simulink model "es3_sim"  (Simulink 7.5)
settings: Solver=ode45  StartTime=0.0  StopTime=10.0  RelTol=1e-3
values from neighbouring files (symbols this model uses):
  e_ = 0.1    [es3.m]
  epsilon1 = 40    [es3.m]
  epsilon2 = 10    [es3.m]
  k1 = 800    [es3.m]
  p = 0.2    [es3.m]
libraries: simulink x1
settings Model: Creator=Koldar  LastModifiedBy=ceco-sciallo

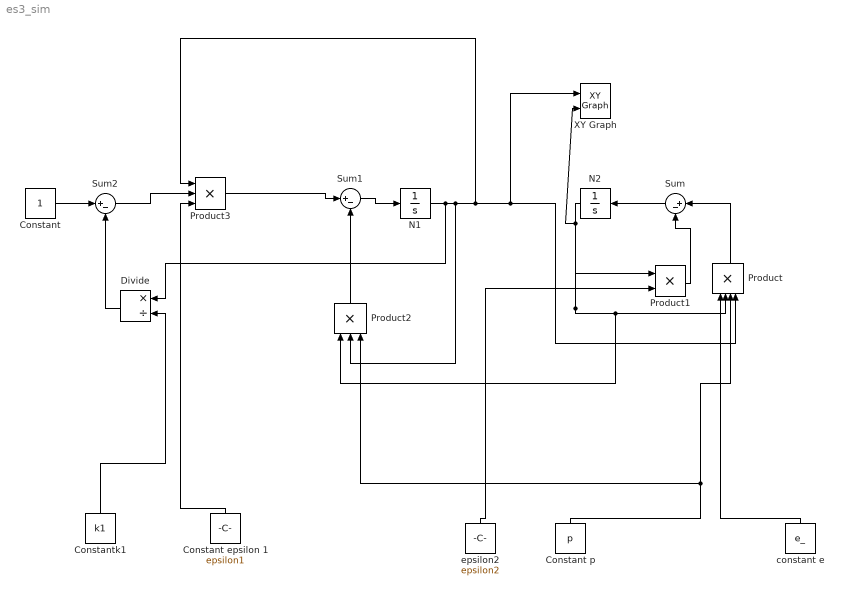
== system es3_sim ==
  Constant : Constant  OutDataType=fixdt(1, 16)  OutScaling=2^0
  Constant epsilon 1 : Constant  Value=epsilon1  OutDataType=fixdt(1, 16)  OutScaling=2^0
  Constant p : Constant  Value=p  OutDataType=fixdt(1, 16)  OutScaling=2^0
  Constantk1 : Constant  Value=k1  OutDataType=fixdt(1, 16)  OutScaling=2^0
  Divide : Product  Inputs=*/  OutDataType=fixdt(1, 16)  OutScaling=2^-10
  N1 : Integrator  InitialCondition=25
  N2 : Integrator  InitialCondition=10
  Product : Product  Inputs=4  OutDataType=fixdt(1, 16)  OutScaling=2^0  RndMeth=Zero
  Product1 : Product  OutDataType=fixdt(1, 16)  OutScaling=2^0  RndMeth=Zero
  Product2 : Product  Inputs=3  OutDataType=fixdt(1, 16)  OutScaling=2^0  RndMeth=Zero
  Product3 : Product  Inputs=3  OutDataType=fixdt(1, 16)  OutScaling=2^0  RndMeth=Zero
  Sum : Sum  Inputs=|+-  OutDataType=fixdt(1, 16)  OutScaling=2^0
  Sum1 : Sum  Inputs=|+-  OutDataType=fixdt(1, 16)  OutScaling=2^0
  Sum2 : Sum  Inputs=|+-  OutDataType=fixdt(1, 16)  OutScaling=2^0
  XY Graph : simulink/Sinks/XY Graph  SystemSampleTime=-1  xmin=0  xmax=100  ymin=0  ymax=100  st=-1
  constant e : Constant  Value=e_  OutDataType=fixdt(1, 16)  OutScaling=2^0
  epsilon2 : Constant  Value=epsilon2  OutDataType=fixdt(1, 16)  OutScaling=2^0
  wires:
  constant e/1 -> Product/1
  Constant p/1 -> Product/3, Product2/3
  N2/1 -> Product1/1, Product/2, Product2/1, XY Graph/2
  N1/1 -> Product2/2, Product3/1, Product/4, XY Graph/1, Divide/1
  Product/1 -> Sum/1
  epsilon2/1 -> Product1/2
  Product1/1 -> Sum/2
  Sum/1 -> N2/1
  Product2/1 -> Sum1/2
  Product3/1 -> Sum1/1
  Sum1/1 -> N1/1
  Constant epsilon 1/1 -> Product3/3
  Constant/1 -> Sum2/1
  Divide/1 -> Sum2/2
  Constantk1/1 -> Divide/2
  Sum2/1 -> Product3/2
